simulink model "SDP_only_Dynamics_test"  (R2024b)
settings: Solver=ode45  StartTime=0.0  StopTime=1800
values from neighbouring files (symbols this model uses):
  Cross_section_area = 0.01    [initialize_satellite_simulation.m]
  d = v_b' * w - cos_th    [cvx_sdp.m]    (also in initialize_satellite_simulation.m = 0.8; solveSDPControl.m)
  delta_t = 0.1    [initialize_satellite_simulation.m]
  finalAngularVelocity = [0; 0; 0]    [initialize_satellite_simulation.m]
  finalAttitude = [cosd(90/2); 0; 0; sind(90/2)]    [initialize_satellite_simulation.m]
  J = diag([Jxx, Jxx, Jxx])    [calculateInertiaTensor.m]    (also in initialize_satellite_simulation.m = calculateInertiaTensor(mass, sideLength); solveSDPControl.m = reshape(u(9:17), 3, 3))
  J2 = J(2,2)    [cvx_sdp.m]
  k = 0.32    [initialize_satellite_simulation.m]
  mass = 1.33    [initialize_satellite_simulation.m]
  theta_min = 50 * (pi / 180)    (= 0.872664625997)    [initialize_satellite_simulation.m]
  v_b = [sin(theta_min); 0; cos(theta_min)]    [initialize_satellite_simulation.m]    (also in solveSDPControl.m = u(4:6))
  w = [0; 0; 1]    [initialize_satellite_simulation.m]    (also in solveSDPControl.m = u(1:3))
undefined symbols (not defined in the file or in its folder): compute_drag
libraries: simulink x5, aerolibutil x4, simulink_extras x1, aerolibgravity2 x1
settings Model: VariantFading=off  LastModifiedBy=shavykashyap
settings SolverCC: ZeroCrossAlgorithm=Adaptive
settings DataIOCC: Refine=2
settings DebuggingCC: SignalInfNanChecking=error  MaskedZcDiagnostic=none  IgnoredZcDiagnostic=none  CheckMatrixSingularityMsg=error

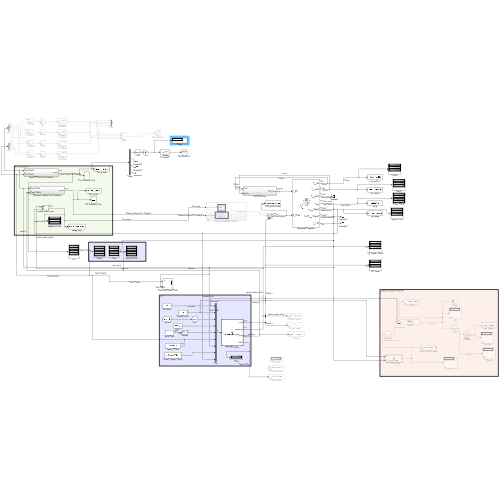
[thumbnail: Simulink's stored preview of the top-level diagram]
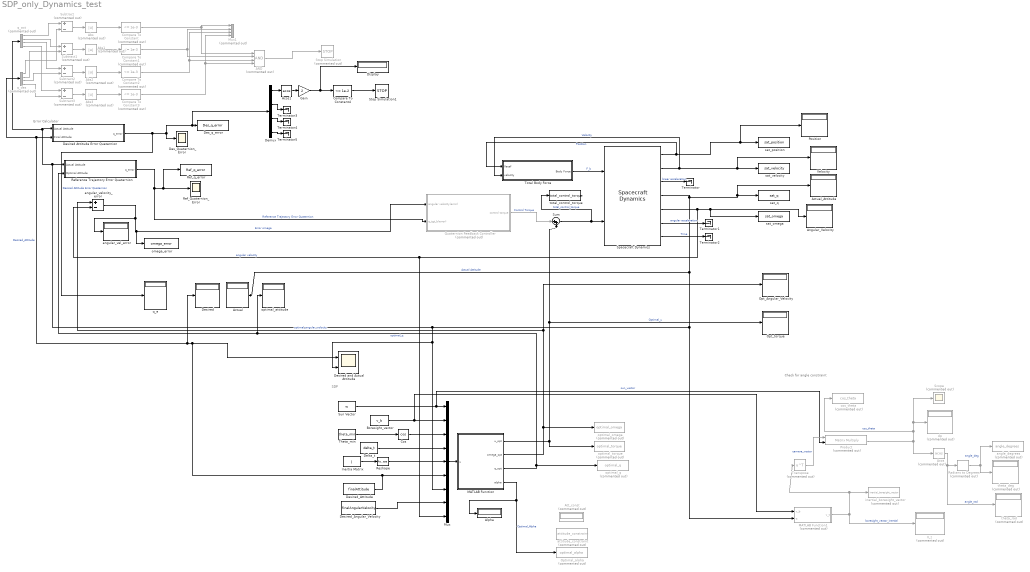
== system SDP_only_Dynamics_test ==
  note: Check for angle constraint
  note: Error Calculator
  note: SDP
  AND : Logic  Commented=on  Inputs=4  IconShape=distinctive  AllPortsSameDT=off  OutDataTypeStr=boolean
  Abs{,1..3} (4 alike) : Abs  Commented=on  SaturateOnIntegerOverflow=off
  Acos : Trigonometry  Commented=on  Operator=acos  RemoveProtectionAgainstOutOfRangeInput=on
  Acos1 : Trigonometry  Operator=acos
  Actual : Display
  Actual_Attitude : Display
  Alpha : Display
  "Angular_Velocity " : Display
  Att_const : Display  Commented=on
  Boresight_vector : Constant  Value=v_b
  Compare To Constant{,1..3} (4 alike) : simulink/Logic and Bit Operations/Compare To Constant  Commented=on  relop=<=  const=1e-3  OutDataTypeStr=boolean
  Compare To Constant4 : simulink/Logic and Bit Operations/Compare To Constant  relop=<=  const=1e-2  OutDataTypeStr=boolean
  Cos : Trigonometry  Operator=cos
  Delta_t : Constant  Value=delta_t
  Demux : Demux
  Des_Quaternion_Error : Scope
  Des_q_error : ToWorkspace  VariableName=Des_q_error  SaveFormat=Timeseries  SampleTime=-1
  Desired : Display
  Desired Attitude Error Quaternion : Subsystem
  Desired and Actual Attitude : Scope  NumInputPorts=2
  Desired_Angular_Velocity : Constant  Value=finalAngularVelocity
  Desired_Attitude : Constant  Value=finalAttitude
  Display : Display
  Gain : Gain  Gain=2
  "Inertia Matrix " : Constant  Value=J
  MATLAB Function : MATLAB Function  TreatAsAtomicUnit=on
  MATLAB Function1 : MATLAB Function  Commented=on  TreatAsAtomicUnit=on
  Mux : Mux  Inputs=9
  Mux1 : Mux  Commented=on
  Opt_Angular_Velocity : Display
  Opt_torque : Display
  Optimal_alpha : ToWorkspace  Commented=on  VariableName=optimal_alpha  SaveFormat=Timeseries  SampleTime=-1
  Position : Display
  Product : Product  Commented=on  Multiplication=Matrix(*)
  "Quaternion Feedback Controller " : Subsystem  Commented=on
  Radians to Degrees : simulink_extras/Transformations/Radians to Degrees  Commented=on
  Ref_Quaternion_Error : Scope
  Ref_q_error : ToWorkspace  VariableName=Ref_q_error  SaveFormat=Timeseries  SampleTime=-1
  Reference Trajectory Error Quaternion : Subsystem
  Reshape : Reshape
  Scope : Scope  Commented=on
  Spacecraft Dynamics : SpacecraftDynamics  outputAccel=on  mass=mass  inertia=J  stateFormatNum=ICRF state vector  inertialPosition=initialPosition  inertialVelocity=initialVelocity  attitude=initialAttitude  attitudeRate=initialAngularVelocity  outputAngAccel=on  gravityModel=Oblate ellipsoid (J2)  useDrag=on  useSRP=on
  Stop Simulation : Stop  Commented=on
  Stop Simulation1 : Stop
  Subtract{,1..3} (4 alike) : Sum  Commented=on  Inputs=+-
  Sum : Sum  Inputs=|++
  "Sun Vector " : Constant  Value=w
  Terminator{,1..5} (6 alike) : Terminator
  Theta_min : Constant  Value=theta_min
  "Total Body Force " : Subsystem
  Transpose : Math  Commented=on  Operator=transpose
  V_t : Display  Commented=on
  Velocity : Display
  angle_degrees : ToWorkspace  Commented=on  VariableName=angle_degrees  SaveFormat=Timeseries  SampleTime=-1
  angular_vel_error : Display
  angular_velocity_error : Sum  Inputs=+-
  attitude_constraint : ToWorkspace  Commented=on  VariableName=attitude_constraint  SaveFormat=Timeseries  SampleTime=-1
  cos_theta : ToWorkspace  Commented=on  VariableName=cos_theta  SaveFormat=Timeseries  SampleTime=-1
  dp : Display  Commented=on
  inertial_boresight_vector : ToWorkspace  Commented=on  VariableName=inertial_boresight_vector  SaveFormat=Timeseries  SampleTime=-1
  omega_error : ToWorkspace  VariableName=omega_error  SaveFormat=Timeseries  SampleTime=-1
  optimal_attitude : Display
  optimal_omega : ToWorkspace  Commented=on  VariableName=optimal_omega  SaveFormat=Timeseries  SampleTime=-1
  optimal_q : ToWorkspace  Commented=on  VariableName=optimal_q  SaveFormat=Timeseries  SampleTime=-1
  optimal_torque : ToWorkspace  Commented=on  VariableName=optimal_torque  SaveFormat=Timeseries  SampleTime=-1
  q_act : Demux  Commented=on
  q_des : Demux  Commented=on
  q_e : Display
  sat_omega : ToWorkspace  VariableName=sat_omega  SaveFormat=Timeseries  SampleTime=-1
  sat_position : ToWorkspace  VariableName=sat_position  SaveFormat=Timeseries  SampleTime=-1
  sat_q : ToWorkspace  VariableName=sat_q  SaveFormat=Timeseries  SampleTime=-1
  sat_velocity : ToWorkspace  VariableName=sat_velocity  SaveFormat=Timeseries  SampleTime=-1
  theta_deg : Display  Commented=on
  theta_rad : Display  Commented=on
  total_control_torque : ToWorkspace  VariableName=total_control_torque  SaveFormat=Timeseries  SampleTime=-1
  wires:
  Spacecraft Dynamics/1 -> "Total Body Force "/1(Xecef), Position/1, sat_position/1  "Position"
  Spacecraft Dynamics/2 -> "Total Body Force "/2(velocity), Velocity/1, sat_velocity/1  "Velocity"
  Spacecraft Dynamics/4 -> Reference Trajectory Error Quaternion/1(Actual Attitude), q_act/1, Desired Attitude Error Quaternion/1(Actual Attitude), Mux/7, Desired and Actual Attitude/2, MATLAB Function1/2(q), Actual/1, Actual_Attitude/1, sat_q/1  "Actual Attitude"
  Spacecraft Dynamics/5 -> Mux/9, angular_velocity_error/2, "Angular_Velocity "/1, sat_omega/1  "angular velocity"
  "Quaternion Feedback Controller "/1(control torque) -> Sum/1  "Control Torque"
  Desired_Attitude/1 -> Desired/1, Desired Attitude Error Quaternion/2(Final Attitude), q_des/1, Desired and Actual Attitude/1, Mux/6  "Desired_Attitude"
  Spacecraft Dynamics/6 -> Terminator1/1  "angular acceleration"
  Spacecraft Dynamics/7 -> Terminator2/1  "Time"
  Spacecraft Dynamics/3 -> Terminator/1  "linear acceleration"
  "Total Body Force "/1(Body Force) -> Spacecraft Dynamics/1  "F_b"
  Sum/1 -> total_control_torque/1, Spacecraft Dynamics/2  "total_control_torque"
  MATLAB Function/1(u_opt) -> Sum/2, Opt_torque/1, optimal_torque/1  "Optimal_u"
  Reference Trajectory Error Quaternion/1(q_error) -> Ref_q_error/1, Ref_Quaternion_Error/1, "Quaternion Feedback Controller "/2(q_tgt_b(error))  "Reference Trajectory Error Quaternion"
  MATLAB Function/3(q_opt) -> optimal_attitude/1, Reference Trajectory Error Quaternion/2(Optimal Attitude), optimal_q/1  "optimal_q"
  "Sun Vector "/1 -> Product/2, Mux/1  "sun_vector"
  Theta_min/1 -> Cos/1
  Delta_t/1 -> Mux/4
  "Inertia Matrix "/1 -> Reshape/1
  Desired_Angular_Velocity/1 -> Mux/8
  Mux/1 -> MATLAB Function/1(u)
  Reshape/1 -> Mux/5
  MATLAB Function/2(omega_opt) -> Opt_Angular_Velocity/1, angular_velocity_error/1, optimal_omega/1  "optimal_angular_velocity"
  Cos/1 -> Mux/3
  angular_velocity_error/1 -> "Quaternion Feedback Controller "/1(angular velocity(error)), omega_error/1, angular_vel_error/1  "Error omega"
  Boresight_vector/1 -> MATLAB Function1/1(v_b), Mux/2
  MATLAB Function1/1(v_t) -> V_t/1, Transpose/1, inertial_boresight_vector/1  "boresight_vector_inertial"
  Acos/1 -> theta_rad/1, Radians to Degrees/1  "angle_rad"
  Radians to Degrees/1 -> theta_deg/1, angle_degrees/1  "angle_deg"
  Transpose/1 -> Product/1  "camera_vector"
  Product/1 -> Acos/1, Scope/1, dp/1, cos_theta/1  "cos_theta"
  MATLAB Function/4(alpha) -> Optimal_alpha/1, Alpha/1  "Optimal_Alpha"
  Desired Attitude Error Quaternion/1(q_error) -> q_e/1, Des_Quaternion_Error/1, Demux/1, Des_q_error/1  "Desired Attitude Error Quaternion"
  AND/1 -> Stop Simulation/1
  q_act/1 -> Subtract/1
  q_des/1 -> Subtract/2
  q_act/2 -> Subtract1/1
  q_act/3 -> Subtract2/1
  q_act/4 -> Subtract3/1
  q_des/2 -> Subtract1/2
  q_des/3 -> Subtract2/2
  q_des/4 -> Subtract3/2
  Subtract/1 -> Abs/1
  Subtract1/1 -> Abs1/1
  Subtract2/1 -> Abs2/1
  Subtract3/1 -> Abs3/1
  Abs/1 -> Compare To Constant/1
  Abs1/1 -> Compare To Constant1/1
  Abs2/1 -> Compare To Constant2/1
  Abs3/1 -> Compare To Constant3/1
  Compare To Constant/1 -> Mux1/1, AND/1
  Compare To Constant1/1 -> Mux1/2, AND/2
  Compare To Constant2/1 -> Mux1/3, AND/3
  Compare To Constant3/1 -> Mux1/4, AND/4
  Demux/1 -> Acos1/1
  Demux/2 -> Terminator3/1
  Demux/3 -> Terminator4/1
  Demux/4 -> Terminator5/1
  Acos1/1 -> Gain/1
  Gain/1 -> Display/1, Compare To Constant4/1
  Compare To Constant4/1 -> Stop Simulation1/1

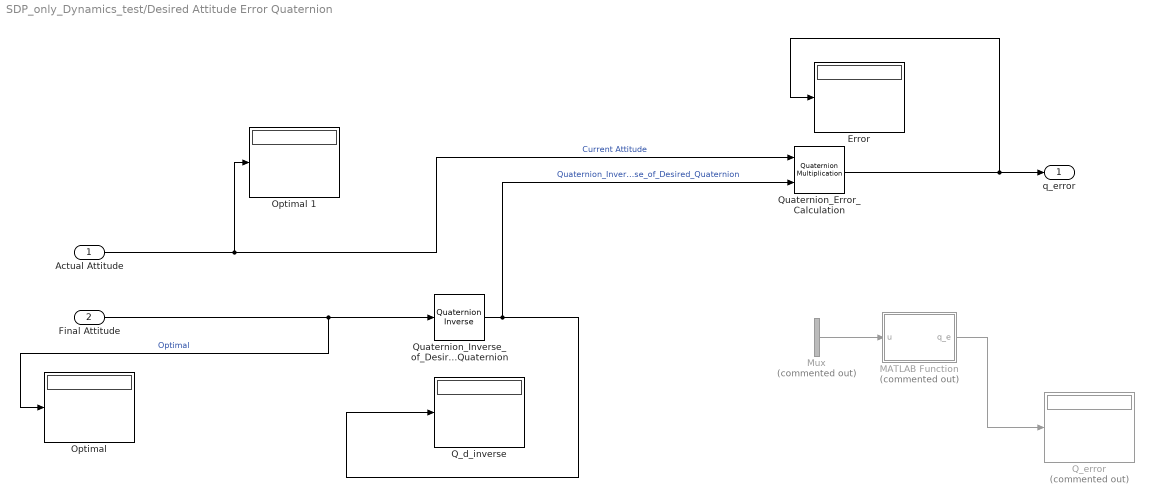
== system SDP_only_Dynamics_test/Desired Attitude Error Quaternion ==
  Actual Attitude : Inport
  Final Attitude : Inport  Port=2
  Error : Display
  MATLAB Function : MATLAB Function  Commented=on  TreatAsAtomicUnit=on
  Mux : Mux  Commented=on  Inputs=2
  "Optimal " : Display
  Optimal 1 : Display
  Q_d_inverse : Display
  Q_error : Display  Commented=on
  Quaternion_Error_Calculation : aerolibutil/Quaternion Multiplication
  Quaternion_Inverse_of_Desired_Quaternion : aerolibutil/Quaternion Inverse
  q_error : Outport
  wires:
  Actual Attitude/1 -> Optimal 1/1, Quaternion_Error_Calculation/1  "Current Attitude"
  Quaternion_Inverse_of_Desired_Quaternion/1 -> Quaternion_Error_Calculation/2, Q_d_inverse/1  "Quaternion_Inverse_of_Desired_Quaternion"
  Quaternion_Error_Calculation/1 -> q_error/1, Error/1
  Final Attitude/1 -> Quaternion_Inverse_of_Desired_Quaternion/1, "Optimal "/1  "Optimal"
  Mux/1 -> MATLAB Function/1(u)
  MATLAB Function/1(q_e) -> Q_error/1

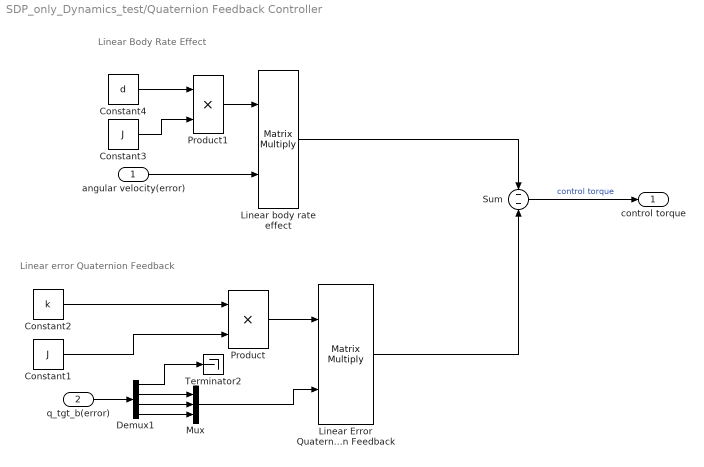
== system SDP_only_Dynamics_test/Quaternion Feedback Controller  ==
  note: Linear error Quaternion Feedback
  note: Linear Body Rate Effect
  angular velocity(error) : Inport
  q_tgt_b(error) : Inport  Port=2
  Constant1 : Constant  Value=J
  Constant2 : Constant  Value=k
  Constant3 : Constant  Value=J
  Constant4 : Constant  Value=d
  Demux1 : Demux
  Linear Error Quaternion Feedback : Product  Multiplication=Matrix(*)
  Linear body rate effect : Product  Multiplication=Matrix(*)
  Mux : Mux  Inputs=3
  Product : Product
  Product1 : Product
  Sum : Sum  Inputs=--
  Terminator2 : Terminator
  control torque : Outport
  wires:
  Linear body rate effect/1 -> Sum/1
  Mux/1 -> Linear Error Quaternion Feedback/2
  angular velocity(error)/1 -> Linear body rate effect/2
  Demux1/1 -> Terminator2/1
  Constant1/1 -> Product/2
  Linear Error Quaternion Feedback/1 -> Sum/2
  Demux1/4 -> Mux/3
  Constant2/1 -> Product/1
  Demux1/2 -> Mux/1
  Demux1/3 -> Mux/2
  Constant3/1 -> Product1/2
  q_tgt_b(error)/1 -> Demux1/1
  Sum/1 -> control torque/1  "control torque"
  Constant4/1 -> Product1/1
  Product/1 -> Linear Error Quaternion Feedback/1
  Product1/1 -> Linear body rate effect/1

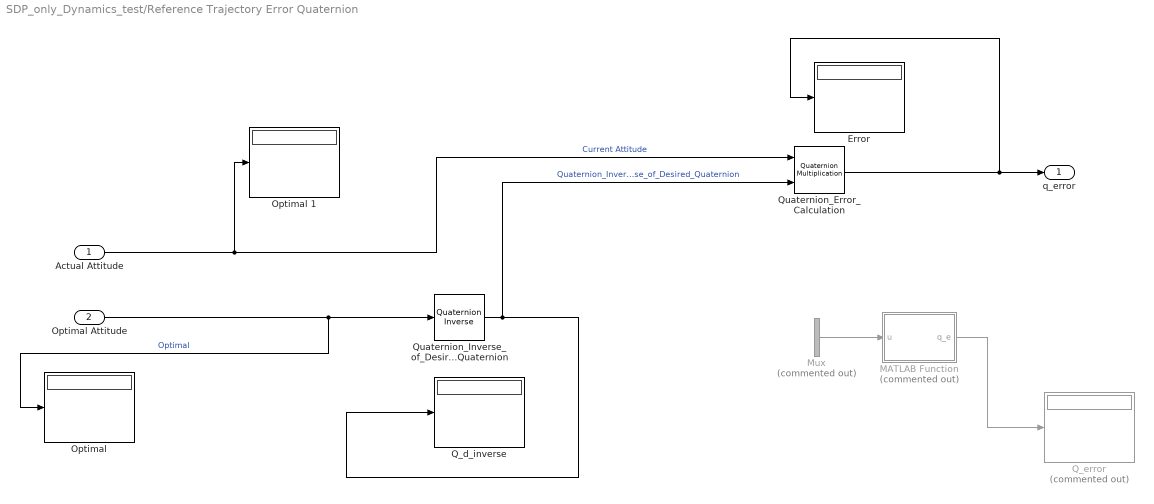
== system SDP_only_Dynamics_test/Reference Trajectory Error Quaternion ==
  Actual Attitude : Inport
  Optimal Attitude : Inport  Port=2
  Error : Display
  MATLAB Function : MATLAB Function  Commented=on  TreatAsAtomicUnit=on
  Mux : Mux  Commented=on  Inputs=2
  "Optimal " : Display
  Optimal 1 : Display
  Q_d_inverse : Display
  Q_error : Display  Commented=on
  Quaternion_Error_Calculation : aerolibutil/Quaternion Multiplication
  Quaternion_Inverse_of_Desired_Quaternion : aerolibutil/Quaternion Inverse
  q_error : Outport
  wires:
  Actual Attitude/1 -> Optimal 1/1, Quaternion_Error_Calculation/1  "Current Attitude"
  Quaternion_Inverse_of_Desired_Quaternion/1 -> Quaternion_Error_Calculation/2, Q_d_inverse/1  "Quaternion_Inverse_of_Desired_Quaternion"
  Quaternion_Error_Calculation/1 -> q_error/1, Error/1
  Optimal Attitude/1 -> Quaternion_Inverse_of_Desired_Quaternion/1, "Optimal "/1  "Optimal"
  Mux/1 -> MATLAB Function/1(u)
  MATLAB Function/1(q_e) -> Q_error/1

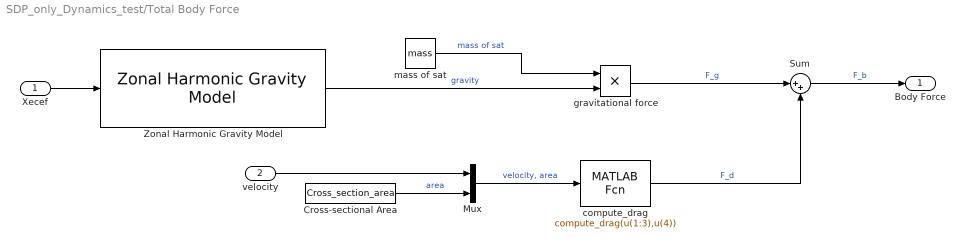
== system SDP_only_Dynamics_test/Total Body Force  ==
  Xecef : Inport
  velocity : Inport  Port=2
  Cross-sectional Area : Constant  Value=Cross_section_area
  Mux : Mux  Inputs=2
  Sum : Sum  Inputs=|++
  Zonal Harmonic Gravity Model : aerolibgravity2/Zonal Harmonic Gravity Model  units=Metric (MKS)  degree=4  action=Warning  ptype=Earth  R=6378136.3  GM=398600441500000  jvalue=[1.0826269e-03 -2.5323000e-06 -1.6204000e-06]
  compute_drag : MATLABFcn  MATLABFcn=compute_drag(u(1:3),u(4))
  gravitational force : Product
  mass of sat : Constant  Value=mass
  Body Force : Outport
  wires:
  mass of sat/1 -> gravitational force/1  "mass of sat"
  compute_drag/1 -> Sum/2  "F_d"
  Mux/1 -> compute_drag/1  "velocity, area"
  Cross-sectional Area/1 -> Mux/2  "area"
  gravitational force/1 -> Sum/1  "F_g"
  Zonal Harmonic Gravity Model/1 -> gravitational force/2  "gravity"
  Xecef/1 -> Zonal Harmonic Gravity Model/1
  Sum/1 -> Body Force/1  "F_b"
  velocity/1 -> Mux/1

== matlab function SDP_only_Dynamics_test/Reference Trajectory Error Quaternion/MATLAB Function ==
  data: u input; q_e output
function q_e = quaternionError(u)
    % quaternionError: Computes the quaternion error between two quaternions.
    % 
    % INPUTS:
    %   q_d - Desired quaternion (commanded attitude) [4x1 column vector]
    %   q   - Current quaternion (actual attitude) [4x1 column vector]
    %
    % OUTPUT:
    %   q_e - Quaternion error q_e = q * q_d^(-1) [4x1 column vector]

    % Extracting inputs that are in the form [a;
    %                                         b;
    %                                         c;
    %                                         d];
    q_d = u(1:4);
    q = u(5:8);

    % Correcting the dimensions for  
    % q_d = q_d';
    % q = q';

    % % Compute the conjugate of q_d (negate vector part, keep scalar unchanged)
    % q_d_conj = [q_d(1); -q_d(2:4)];

    % Compute the inverse of q_d (for unit quaternions, this is just its conjugate)
    q_d_inv = quatinv(q_d');    % Using the transpose , since the quatinv function requires [1x4] inputs 
    q_d_inv = q_d_inv';         % taking the transpose of the inverse to make the dimensions [4x1] which is required for the 

    % Compute quaternion error: q_e = q * q_d_inv (Hamilton product)
    % Quaternion multiplication formula:
    % Scalar part:  q_e(1) = q0 * p0 - (q_v • p_v)
    % Vector part:  q_e(2:4) = q0 * p_v + p0 * q_v - (q_v × p_v)
    q_e = [ q(1) * q_d_inv(1) - dot(q(2:4), q_d_inv(2:4));   % Scalar part
            q_d_inv(1) * q(2:4) + q(1) * q_d_inv(2:4) - cross(q(2:4), q_d_inv(2:4)) ]; % Vector part

    % q_e = q_e';
    % % Normalize quaternion error to ensure it remains a unit quaternion
    q_e = q_e / norm(q_e);
    % q_e = q_e';

end

== matlab function SDP_only_Dynamics_test/MATLAB Function ==
  data: u_opt output; u input; omega_opt output; q_opt output; alpha output
function [u_opt,omega_opt, q_opt,    alpha]  = solveSDPWrapper(u)
    % Declare function as extrinsic for Simulink
    coder.extrinsic('solveSDPControl'); 

    % Define a placeholder output (to prevent Simulink errors)
    u_opt = zeros(3,1);
    omega_opt = zeros(3,1);
    q_opt = zeros(4,1);
    alpha = zeros(1,1);
    % att_const = zeros(1,1);

    % Pack inputs into a single vector
    % u = [w; v_b; theta_min; delta_t; J(:); q_d; q; omega_N; omega; N];

    % Call the original SDP solver
    [u_opt, omega_opt, q_opt, alpha] = solveSDPControl(u);

end

% 
% function [u_opt, omega_opt, q_opt, alpha] = solveSDPWrapper(u_vec)
% % Wrapper that calls the cached SDP optimiser from Simulink
% 
% % Tell Simulink these functions run in the MATLAB interpreter
% coder.extrinsic('evalin');
% coder.extrinsic('solveSDPControl_cached');
% coder.extrinsic('yalmiperror');
% 
% % Grab constant struct 'par' from base workspace only once
% persistent par isInit
% if isempty(isInit)
%     par = evalin('base','par');   % OK, evalin is extrinsic
%     isInit    = true;
% end
% 
% % Pre‑allocate fixed‑size outputs (required for code‑gen)
% u_opt     = zeros(3,1);   % 3×1 torque
% omega_opt = zeros(3,1);   % 3×1 body rates
% q_opt     = zeros(4,1);   % 4×1 quaternion
% alpha     = 0;            % scalar slack
% 
% % Un‑pack the time‑varying states from the 31×1 vector
% %   (first 4 elements = quaternion, next 3 = body‑rates)
% q_now     = u_vec(1:4);     % 4×1 current quaternion
% omega_now = u_vec(5:7);     % 3×1 current angular rate
% 
% % Call the cached SDP solver (extrinsic)
% [uu, om, qq, aa] = solveSDPControl_cached(par, q_now,omega_now);
% 
% %------------------------------------------------------------------
% % NaN / Inf guard + torque saturation  (same limits as plant)
% % if any(~isfinite([uu; om; qq; aa]))
% %     % Show solver status code in readable form
% %     disp(['>>> SDP issue: ', yalmiperror(aa)]);
% %     uu = zeros(3,1);
% %     om = zeros(3,1);
% %     qq = [1;0;0;0];
% %     aa = 0;
% % end
% 
% % uu = min(max(uu, -2e-4),  2e-4);        % actuator limits
% % qq = qq / max(norm(qq), 1e-12);         % ensure unit quaternion
% 
% %------------------------------------------------------------------
% u_opt     = uu;
% omega_opt = om;
% q_opt     = qq;
% alpha     = aa;
% end

== matlab function SDP_only_Dynamics_test/MATLAB Function1 ==
  data: v_b input; v_t output; q input
function v_t = rotateVector(v_b, q)
% rotateVector Rotates a body-frame vector into the inertial frame
%              using a quaternion.
%
%   v_t = rotateVector(v_b, w, q) returns the inertial frame vector v_t,
%   given the body-frame vector v_b, an inertial vector w (for reference),
%   and the quaternion q.
%
%   Inputs:
%     v_b : 3x1 vector in the body frame (e.g., the boresight)
%     w   : 3x1 reference vector in the inertial frame (e.g., the sun vector)
%           (Note: In this function, w is not used in the rotation, but is
%           provided for consistency with your formulation.)
%     q   : 4x1 quaternion [q1; q2; q3; q4], where q1:q3 is the vector part,
%           and q4 is the scalar part.
%
%   Output:
%     v_t : 3x1 vector in the inertial frame, after applying the quaternion rotation.
%
%   The rotation is computed using the formula:
%
%     v_t = v_b - 2*(q_vec' * q_vec)*v_b + 2*(q_vec' * v_b)*q_vec - 2*q_sca*cross(v_b, q_vec)
%
%   where q_vec = [q1; q2; q3] and q_sca = q4.


    % Extract the vector and scalar parts of the quaternion
    q_vec = q(2:4);
    q_sca = q(1);

    % Apply the rotation formula
    v_t = v_b - 2*(q_vec' * q_vec)*v_b + 2*(q_vec' * v_b)*q_vec - 2*q_sca*cross(v_b, q_vec);
end

== matlab function SDP_only_Dynamics_test/Desired Attitude Error Quaternion/MATLAB Function ==
  data: u input; q_e output
function q_e = quaternionError(u)
    % quaternionError: Computes the quaternion error between two quaternions.
    % 
    % INPUTS:
    %   q_d - Desired quaternion (commanded attitude) [4x1 column vector]
    %   q   - Current quaternion (actual attitude) [4x1 column vector]
    %
    % OUTPUT:
    %   q_e - Quaternion error q_e = q * q_d^(-1) [4x1 column vector]

    % Extracting inputs that are in the form [a;
    %                                         b;
    %                                         c;
    %                                         d];
    q_d = u(1:4);
    q = u(5:8);

    % Correcting the dimensions for  
    % q_d = q_d';
    % q = q';

    % % Compute the conjugate of q_d (negate vector part, keep scalar unchanged)
    % q_d_conj = [q_d(1); -q_d(2:4)];

    % Compute the inverse of q_d (for unit quaternions, this is just its conjugate)
    q_d_inv = quatinv(q_d');    % Using the transpose , since the quatinv function requires [1x4] inputs 
    q_d_inv = q_d_inv';         % taking the transpose of the inverse to make the dimensions [4x1] which is required for the 

    % Compute quaternion error: q_e = q * q_d_inv (Hamilton product)
    % Quaternion multiplication formula:
    % Scalar part:  q_e(1) = q0 * p0 - (q_v • p_v)
    % Vector part:  q_e(2:4) = q0 * p_v + p0 * q_v - (q_v × p_v)
    q_e = [ q(1) * q_d_inv(1) - dot(q(2:4), q_d_inv(2:4));   % Scalar part
            q_d_inv(1) * q(2:4) + q(1) * q_d_inv(2:4) - cross(q(2:4), q_d_inv(2:4)) ]; % Vector part

    % q_e = q_e';
    % % Normalize quaternion error to ensure it remains a unit quaternion
    q_e = q_e / norm(q_e);
    % q_e = q_e';

end
